simulink model "pack_2s1p_example"  (R2022a)
settings: Solver=VariableStepAuto  StartTime=0.0  StopTime=param.end_time  RelTol=1e-3
values from neighbouring files (symbols this model uses):
  param = table2struct(readtable('settings.csv'))    [run_pybamm_pack.m]
libraries: fl_lib x13, spsParallelRLCBranchLib x8, nesl_utility x5, spsCurrentMeasurementLib x4, spsVoltageMeasurementLib x3, spsControlledVoltageSourceLib x2, spsVariableResistorLib x2, spsControlledCurrentSourceLib x1, spspowerguiLib x1
settings Model: Creator=tom  LastModifiedBy=Vivian
settings SolverCC: AlgebraicLoopSolver=TrustRegion
settings DebuggingCC: UnconnectedInputMsg=warning  UnconnectedOutputMsg=warning  UnconnectedLineMsg=warning  SFMachineParentedDataDiag=warning
settings RTWCC: DLArmComputeVersion=19.05

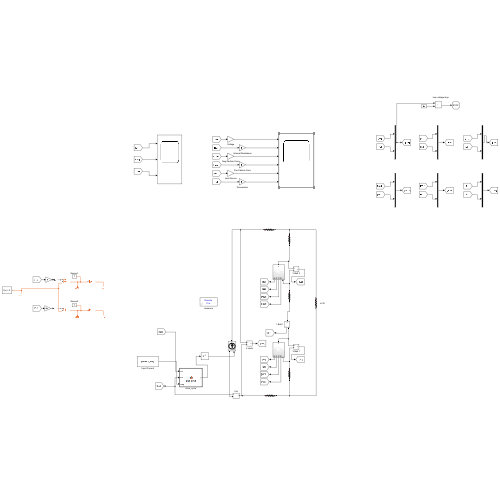
[thumbnail: Simulink's stored preview of the top-level diagram]
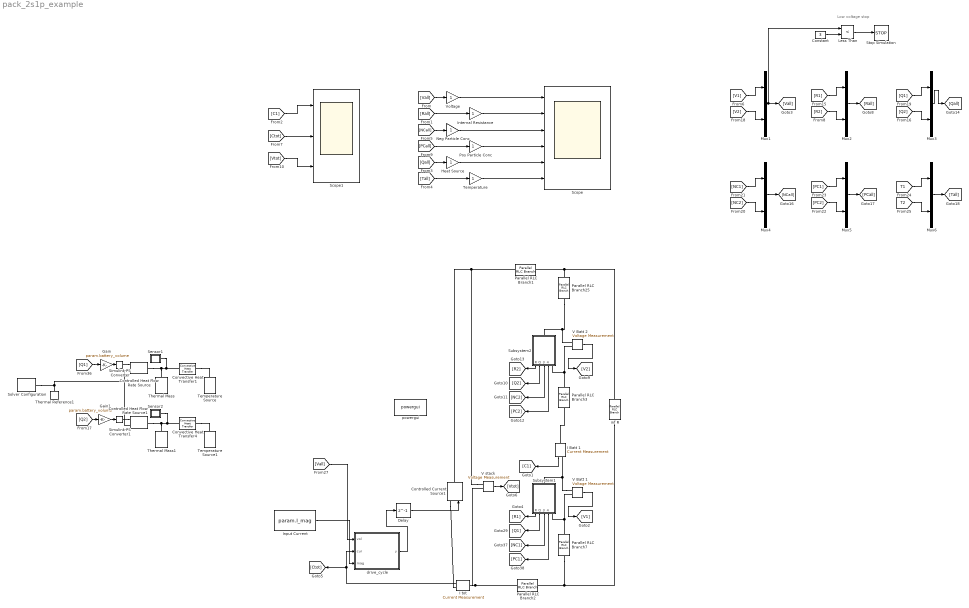
== system pack_2s1p_example ==
  note: Low voltage stop
  Constant : Constant  Value=3
  Controlled Current Source1 : spsControlledCurrentSourceLib/Controlled Current Source  Initialize=on  Source_Type=DC  Amplitude=0  Phase=0  Frequency=0  Measurements=None
  Controlled Heat Flow Rate Source : fl_lib/Thermal/Thermal Sources/Controlled Heat Flow Rate Source
      settings: SourceProductBaseCode=PW,SS,VE
  Controlled Heat Flow Rate Source1 : fl_lib/Thermal/Thermal Sources/Controlled Heat Flow Rate Source
      settings: SourceProductBaseCode=PW,SS,VE
  Convective Heat Transfer1 : fl_lib/Thermal/Thermal Elements/Convective Heat Transfer  area=param.cooled_surface_area m^2  heat_tr_coeff=param.cooling_coefficient W/(m^2 * K)  T_specify=off  T_priority=None  T=0 K  T_nominal_specify=off  T_nominal_unit=K  T_nominal_value=1  Q_specify=off  Q_priority=None  Q=0 W  Q_nominal_specify=off  Q_nominal_unit=W  Q_nominal_value=1
      settings: SourceProductBaseCode=PW,SS,VE
  Convective Heat Transfer4 : fl_lib/Thermal/Thermal Elements/Convective Heat Transfer  area=param.cooled_surface_area m^2  heat_tr_coeff=param.cooling_coefficient W/(m^2 * K)  T_specify=off  T_priority=None  T=0 K  T_nominal_specify=off  T_nominal_unit=K  T_nominal_value=1  Q_specify=off  Q_priority=None  Q=0 W  Q_nominal_specify=off  Q_nominal_unit=W  Q_nominal_value=1
      settings: SourceProductBaseCode=PW,SS,VE
  Delay : Delay  DelayLength=1  InitialCondition=param.I_app
  Gain : Gain  Gain=param.battery_volume
  Gain1 : Gain  Gain=param.battery_volume
  Heat Source : Gain
  I Batt 1 : spsCurrentMeasurementLib/Current Measurement  PhasorSimulation=off  OutputType=Complex  PSBequivalent=0
  I tot : spsCurrentMeasurementLib/Current Measurement  PhasorSimulation=off  OutputType=Complex  PSBequivalent=0
  Input Current : Constant  Value=param.I_mag
  Internal Resistance : Gain
  Less Than : RelationalOperator  Operator=<  OutDataTypeStr=boolean  RndMeth=Simplest  InputSameDT=off
  Mux{1..6} (6 alike) : Mux  Inputs=2
  Neg Particle Conc : Gain
  Parallel RLC Branch1 : spsParallelRLCBranchLib/Parallel RLC Branch  LConnTagsString=a  RConnTagsString=__new0  BranchType=R  Resistance=param.R_connect  Inductance=1e-3  SetiL0=off  InitialCurrent=0  Capacitance=1e-6  Setx0=off  InitialVoltage=0  Measurements=None
  Parallel RLC Branch2 : spsParallelRLCBranchLib/Parallel RLC Branch  LConnTagsString=a  RConnTagsString=__new0  BranchType=R  Resistance=param.R_connect  Inductance=1e-3  SetiL0=off  InitialCurrent=0  Capacitance=1e-6  Setx0=off  InitialVoltage=0  Measurements=None
  Parallel RLC Branch25 : spsParallelRLCBranchLib/Parallel RLC Branch  LConnTagsString=a  RConnTagsString=__new0  BranchType=R  Resistance=param.R_series_top  Inductance=1e-3  SetiL0=off  InitialCurrent=0  Capacitance=1e-6  Setx0=off  InitialVoltage=0  Measurements=None
  Parallel RLC Branch3 : spsParallelRLCBranchLib/Parallel RLC Branch  LConnTagsString=a  RConnTagsString=__new0  BranchType=R  Resistance=param.R_series_mid  Inductance=1e-3  SetiL0=off  InitialCurrent=0  Capacitance=1e-6  Setx0=off  InitialVoltage=0  Measurements=None
  Parallel RLC Branch7 : spsParallelRLCBranchLib/Parallel RLC Branch  LConnTagsString=a  RConnTagsString=__new0  BranchType=R  Resistance=param.R_series_bottom  Inductance=1e-3  SetiL0=off  InitialCurrent=0  Capacitance=1e-6  Setx0=off  InitialVoltage=0  Measurements=None
  Pos Particle Conc : Gain
  Scope : Scope  NumInputPorts=6
  Scope1 : Scope  NumInputPorts=3
  Sensor1 : Subsystem
      mask Display: disp('T')
  Sensor2 : Subsystem
      mask Display: disp('T')
  Simulink-PS Converter : nesl_utility/Simulink-PS Converter  PhysicalDomain=network_engine_domain  SubClassName=ps_input  LeftPortType=input  RightPortType=output  PseudoPeriodic=off  Frequencies=[]  NoiseDistribution=none  NoiseParameters=[]  Unit=1  AffineConversion=off  FilteringAndDerivatives=provide  SimscapeFilterOrder=1  InputFilterTimeConstant=0.001  UdotUserProvided=0
      settings: SourceProductBaseCode=SS,PW,VE
  Simulink-PS Converter1 : nesl_utility/Simulink-PS Converter  PhysicalDomain=network_engine_domain  SubClassName=ps_input  LeftPortType=input  RightPortType=output  PseudoPeriodic=off  Frequencies=[]  NoiseDistribution=none  NoiseParameters=[]  Unit=1  AffineConversion=off  FilteringAndDerivatives=provide  SimscapeFilterOrder=1  InputFilterTimeConstant=0.001  UdotUserProvided=0
      settings: SourceProductBaseCode=SS,PW,VE
  Solver Configuration : nesl_utility/Solver Configuration  PhysicalDomain=network_engine_domain  SubClassName=solver  LeftPortType=input  RightPortType=generic  Tones=[]  Harmonics=[]  SimulateNoise=off  Profile=off  UseLocalSampling=off  EnableSwitchedLinearOptims=on  FrequencyDomain=off  UseCCode=off  RelTol=0.001  AbsTol=1e-06  MinStep=1e-09  ToWorkspace=off  RevertToSquareIcSolve=off  NumHomotopyIterations=100  PhasorMode=off  PhasorModeNumHarmonics=1  IndexReductionMethod=DerivativeReplacement  DoDC=off  ResidualTolerance=1e-09  UseLocalSolver=on  LocalSolverChoice=NE_BACKWARD_EULER_ADVANCER  LocalSolverSampleTime=param.dt  DoFixedCost=on  MaxNonlinIter=3  MaxModeIter=2  ComputeImpulses=off  ImpulseIterations=2  LinearAlgebra=auto  LinearAlgebraNumThread=0  EquationFormulation=NE_TIME_EF  DelaysMemoryBudget=1024  AutomaticFiltering=on  FilteringTimeConstant=0.001  PartitionStorageMethod=AS_NEEDED  PartitionMemoryBudget=1024  PartitionMethod=ROBUST
      settings: SourceProductBaseCode=SS,PW,VE
  Stop Simulation : Stop
  Subsystem1 : Subsystem
  Subsystem2 : Subsystem
  Temperature : Gain
  Temperature Source : fl_lib/Thermal/Thermal Sources/Temperature Source  temperature=param.reference_temperature K
      settings: SourceProductBaseCode=PW,SS,VE
  Temperature Source1 : fl_lib/Thermal/Thermal Sources/Temperature Source  temperature=param.reference_temperature K
      settings: SourceProductBaseCode=PW,SS,VE
  Thermal Mass : fl_lib/Thermal/Thermal Elements/Thermal Mass  mass=param.battery_mass kg  sp_heat=param.Cp J/kg/K  T_specify=on  T_priority=High  T=param.reference_temperature K  T_nominal_specify=off  T_nominal_unit=K  T_nominal_value=1  Q_specify=off  Q_priority=None  Q=0 W  Q_nominal_specify=off  Q_nominal_unit=W  Q_nominal_value=1
      settings: SourceProductBaseCode=PW,SS,VE
  Thermal Mass1 : fl_lib/Thermal/Thermal Elements/Thermal Mass  mass=param.battery_mass kg  sp_heat=param.Cp J/kg/K  T_specify=on  T_priority=High  T=param.reference_temperature K  T_nominal_specify=off  T_nominal_unit=K  T_nominal_value=1  Q_specify=off  Q_priority=None  Q=0 W  Q_nominal_specify=off  Q_nominal_unit=W  Q_nominal_value=1
      settings: SourceProductBaseCode=PW,SS,VE
  Thermal Reference1 : fl_lib/Thermal/Thermal Elements/Thermal Reference
      settings: SourceProductBaseCode=PW,SS,VE
  V Batt 1 : spsVoltageMeasurementLib/Voltage Measurement  PhasorSimulation=off  OutputType=Complex  PSBequivalent=0
  V Batt 2 : spsVoltageMeasurementLib/Voltage Measurement  PhasorSimulation=off  OutputType=Complex  PSBequivalent=0
  V stack : spsVoltageMeasurementLib/Voltage Measurement  PhasorSimulation=off  OutputType=Complex  PSBequivalent=0
  Voltage : Gain
  drive_cycle : MATLAB Function  TreatAsAtomicUnit=on
  inf R : spsParallelRLCBranchLib/Parallel RLC Branch  LConnTagsString=a  RConnTagsString=__new0  BranchType=R  Resistance=100000  Inductance=1e-3  SetiL0=off  InitialCurrent=0  Capacitance=1e-6  Setx0=off  InitialVoltage=0  Measurements=None
  powergui : spspowerguiLib/powergui  Priority=1  SimulationMode=Discrete  SampleTime=param.dt  frequency=60  Iterations=50  frequencyindice=0  Pbase=100e6  ErrMax=1e-4  UnitsV=kV  UnitsW=MW  buscounter=0  FunctionMessages=off  echomessages=off  EnableUseOfTLC=off  CurrentSourceSwitches=off  DisableSnubberDevices=off  DisableRonSwitches=off  DisableVfSwitches=off  DisplayEquations=off  AutomaticDiscreteSolvers=off  SolverType=Tustin/Backward Euler (TBE)  Interpol=off  ExternalGateDelay=off  methode=off  Ts=100  x0status=blocks  SPID=on  SwTol=0  HookPort=off  NonlinearTolerance=1e-4  nMaxIteration=100  ContinueOnMaxIteration=off  RestoreLinks=warning  ResistiveCurrentMeasurement=off  Frange=[0:2:500]  Ylog=off  Xlog=on  ShowGrid=off  save=off  variable=ZData  structure=0  ZoomFFT=off  StartTime=0.0  cycles=1  DisplayStyle=1  fundamental=60  FreqAxis=off  MaxFrequency=1000  frequencyindicesteady=1  RmsSteady=1  display=off
  wires:
  Input Current/1 -> drive_cycle/3(mag)
  [Vall] -> drive_cycle/1(vol)
  drive_cycle/1(y) -> Delay/1
  V stack/1 -> [Vtot]
  V Batt 1/1 -> [V1]
  I Batt 1/1 -> [C1]
  Subsystem1/2(Q) -> [Q1]
  Gain/1 -> Simulink-PS Converter/1
  [Q1] -> Gain/1
  [Vall] -> Voltage/1
  [Rall] -> Internal Resistance/1
  [NCall] -> Neg Particle Conc/1
  [PCall] -> Pos Particle Conc/1
  [Qall] -> Heat Source/1
  [Tall] -> Temperature/1
  [V1] -> Mux1/1
  Mux1/1 -> Less Than/1, [Vall]
  I tot/1 -> [Ctot], drive_cycle/2(cur)
  Subsystem1/1(R) -> [R1]
  Subsystem2/1(R) -> [R2]
  Subsystem2/2(Q) -> [Q2]
  V Batt 2/1 -> [V2]
  [Q2] -> Gain1/1
  Gain1/1 -> Simulink-PS Converter1/1
  [V2] -> Mux1/2
  Delay/1 -> Controlled Current Source1/1
  [R2] -> Mux2/2
  Mux2/1 -> [Rall]
  [R1] -> Mux2/1
  [Q2] -> Mux3/2
  Mux3/1 -> [Qall]
  [Q1] -> Mux3/1
  [NC2] -> Mux4/2
  Mux4/1 -> [NCall]
  [NC1] -> Mux4/1
  Mux5/1 -> [PCall]
  [PC2] -> Mux5/2
  [PC1] -> Mux5/1
  [T1] -> Mux6/1
  Mux6/1 -> [Tall]
  [T2] -> Mux6/2
  Voltage/1 -> Scope/1
  Internal Resistance/1 -> Scope/2
  Neg Particle Conc/1 -> Scope/3
  Pos Particle Conc/1 -> Scope/4
  Heat Source/1 -> Scope/5
  Temperature/1 -> Scope/6
  Subsystem2/3(nc) -> [NC2]
  Subsystem2/4(pc) -> [PC2]
  Subsystem1/3(nc) -> [NC1]
  Subsystem1/4(pc) -> [PC1]
  [C1] -> Scope1/1
  [Ctot] -> Scope1/2
  [Vtot] -> Scope1/3
  Less Than/1 -> Stop Simulation/1
  Constant/1 -> Less Than/2
  connections:
  Parallel RLC Branch25/LConn1 -- inf R/LConn1 -- Parallel RLC Branch1/RConn1
  V stack/LConn1 -- Controlled Current Source1/RConn1 -- Parallel RLC Branch1/LConn1
  Subsystem1/RConn1 -- V Batt 1/LConn2 -- Parallel RLC Branch7/LConn1
  V Batt 1/LConn1 -- I Batt 1/RConn1 -- Subsystem1/LConn1
  V stack/LConn2 -- Parallel RLC Branch2/LConn1 -- I tot/LConn1
  Parallel RLC Branch7/RConn1 -- Parallel RLC Branch2/RConn1 -- inf R/RConn1
  Thermal Mass/LConn1 -- Sensor1/LConn1 -- Convective Heat Transfer1/LConn1 -- Controlled Heat Flow Rate Source/LConn1
  Simulink-PS Converter/RConn1 -- Controlled Heat Flow Rate Source/RConn1
  Thermal Reference1/LConn1 -- Solver Configuration/RConn1 -- Controlled Heat Flow Rate Source1/RConn2 -- Controlled Heat Flow Rate Source/RConn2
  Controlled Current Source1/LConn1 -- I tot/RConn1
  Subsystem2/RConn1 -- Parallel RLC Branch3/LConn1 -- V Batt 2/LConn2
  Subsystem2/LConn1 -- Parallel RLC Branch25/RConn1 -- V Batt 2/LConn1
  I Batt 1/LConn1 -- Parallel RLC Branch3/RConn1
  Thermal Mass1/LConn1 -- Sensor2/LConn1 -- Convective Heat Transfer4/LConn1 -- Controlled Heat Flow Rate Source1/LConn1
  Simulink-PS Converter1/RConn1 -- Controlled Heat Flow Rate Source1/RConn1
  Convective Heat Transfer4/RConn1 -- Temperature Source1/LConn1
  Convective Heat Transfer1/RConn1 -- Temperature Source/LConn1

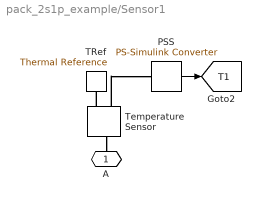
== system pack_2s1p_example/Sensor1 ==
  PSS : nesl_utility/PS-Simulink Converter  PhysicalDomain=network_engine_domain  SubClassName=ps_output  LeftPortType=input  RightPortType=output  PseudoPeriodic=off  Frequencies=[]  VectorFormat=1-D array  Unit=1  AffineConversion=off
      settings: SourceProductBaseCode=SS,PW,VE
  TRef : fl_lib/Thermal/Thermal Elements/Thermal Reference
      settings: SourceProductBaseCode=PW,SS,VE
  Temperature Sensor : fl_lib/Thermal/Thermal Sensors/Temperature Sensor
      settings: SourceProductBaseCode=PW,SS,VE
  A : PMIOPort  Side=Left
  tag scope: T1=global
  wires:
  PSS/1 -> [T1]
  connections:
  Temperature Sensor/RConn2 -- PSS/LConn1
  Temperature Sensor/RConn1 -- TRef/LConn1
  Temperature Sensor/LConn1 -- A/RConn1

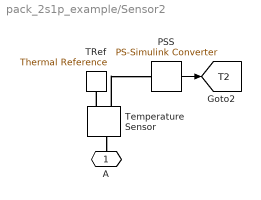
== system pack_2s1p_example/Sensor2 ==
  PSS : nesl_utility/PS-Simulink Converter  PhysicalDomain=network_engine_domain  SubClassName=ps_output  LeftPortType=input  RightPortType=output  PseudoPeriodic=off  Frequencies=[]  VectorFormat=1-D array  Unit=1  AffineConversion=off
      settings: SourceProductBaseCode=SS,PW,VE
  TRef : fl_lib/Thermal/Thermal Elements/Thermal Reference
      settings: SourceProductBaseCode=PW,SS,VE
  Temperature Sensor : fl_lib/Thermal/Thermal Sensors/Temperature Sensor
      settings: SourceProductBaseCode=PW,SS,VE
  A : PMIOPort  Side=Left
  tag scope: T2=global
  wires:
  PSS/1 -> [T2]
  connections:
  Temperature Sensor/LConn1 -- A/RConn1
  Temperature Sensor/RConn1 -- TRef/LConn1
  Temperature Sensor/RConn2 -- PSS/LConn1

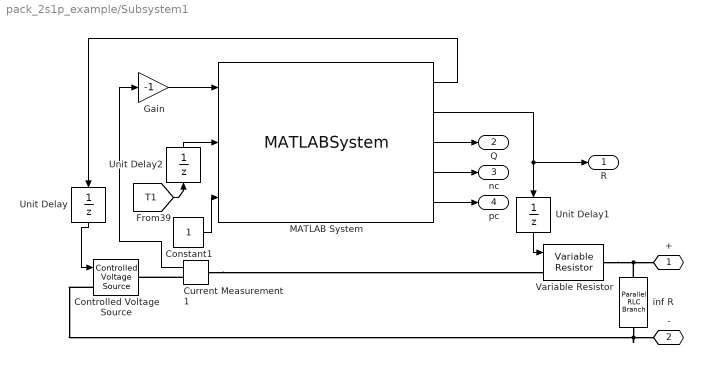
== system pack_2s1p_example/Subsystem1 ==
  Constant1 : Constant
  Controlled Voltage Source : spsControlledVoltageSourceLib/Controlled Voltage Source  Initialize=on  Source_Type=AC  Amplitude=0  Phase=0  Frequency=0  Measurements=None
  Current Measurement1 : spsCurrentMeasurementLib/Current Measurement  PhasorSimulation=off  OutputType=Complex  PSBequivalent=0
  Gain : Gain  Gain=-1
  MATLAB System : MATLABSystem  System=casadi_bat  SimulateUsing=Interpreted execution
      mask Type: casadi_bat
      mask Display:
      | disp('casadi_bat');
      | port_label('input',1,'current');
      | port_label('input',2,'temperature');
      | port_label('input',3,'soc_init');
      | port_label('output',1,'ocp');
      | port_label('output',2,'internal_resistance');
      | port_label('output',3,'heating');
      | port_label('output',4,'neg_conc');
      | port_label('output',5,'pos_conc');
  Unit Delay : UnitDelay  InitialCondition=param.ocv_init  SampleTime=-1  HasFrameUpgradeWarning=on
  Unit Delay1 : UnitDelay  InitialCondition=param.r_int_init  SampleTime=-1  HasFrameUpgradeWarning=on
  Unit Delay2 : UnitDelay  InitialCondition=param.t_init  SampleTime=-1  HasFrameUpgradeWarning=on
  Variable Resistor : spsVariableResistorLib/Variable Resistor  Rabsmin=1e-3
      settings: SourceProductBaseCode=PS
  inf R : spsParallelRLCBranchLib/Parallel RLC Branch  LConnTagsString=a  RConnTagsString=__new0  BranchType=R  Resistance=100000  Inductance=1e-3  SetiL0=off  InitialCurrent=0  Capacitance=1e-6  Setx0=off  InitialVoltage=0  Measurements=None
  + : PMIOPort  Tag=PMCPort  Side=Left
  - : PMIOPort  Tag=PMCPort  Port=2  Side=Right
  R : Outport  VectorParamsAs1DForOutWhenUnconnected=off
  Q : Outport  Port=2  VectorParamsAs1DForOutWhenUnconnected=off
  nc : Outport  Port=3  VectorParamsAs1DForOutWhenUnconnected=off
  pc : Outport  Port=4  VectorParamsAs1DForOutWhenUnconnected=off
  wires:
  Gain/1 -> MATLAB System/1
  MATLAB System/1 -> Unit Delay/1
  Current Measurement1/1 -> Gain/1
  Unit Delay/1 -> Controlled Voltage Source/1
  MATLAB System/2 -> R/1, Unit Delay1/1
  Unit Delay1/1 -> Variable Resistor/1
  MATLAB System/3 -> Q/1
  Unit Delay2/1 -> MATLAB System/2
  [T1] -> Unit Delay2/1
  MATLAB System/5 -> pc/1
  MATLAB System/4 -> nc/1
  Constant1/1 -> MATLAB System/3
  connections:
  Current Measurement1/RConn1 -- Controlled Voltage Source/RConn1
  Controlled Voltage Source/LConn1 -- inf R/RConn1 -- -/RConn1
  Current Measurement1/LConn1 -- Variable Resistor/LConn1
  Variable Resistor/RConn1 -- inf R/LConn1 -- +/RConn1

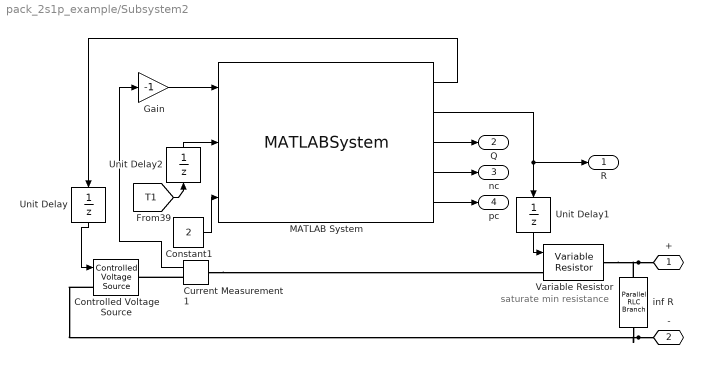
== system pack_2s1p_example/Subsystem2 ==
  note: saturate min resistance
  Constant1 : Constant  Value=2
  Controlled Voltage Source : spsControlledVoltageSourceLib/Controlled Voltage Source  Initialize=on  Source_Type=AC  Amplitude=0  Phase=0  Frequency=0  Measurements=None
  Current Measurement1 : spsCurrentMeasurementLib/Current Measurement  PhasorSimulation=off  OutputType=Complex  PSBequivalent=0
  Gain : Gain  Gain=-1
  MATLAB System : MATLABSystem  System=casadi_bat  SimulateUsing=Interpreted execution
      mask Type: casadi_bat
      mask Display:
      | disp('casadi_bat');
      | port_label('input',1,'current');
      | port_label('input',2,'temperature');
      | port_label('input',3,'soc_init');
      | port_label('output',1,'ocp');
      | port_label('output',2,'internal_resistance');
      | port_label('output',3,'heating');
      | port_label('output',4,'neg_conc');
      | port_label('output',5,'pos_conc');
  Unit Delay : UnitDelay  InitialCondition=param.ocv_init  SampleTime=-1  HasFrameUpgradeWarning=on
  Unit Delay1 : UnitDelay  InitialCondition=param.r_int_init  SampleTime=-1  HasFrameUpgradeWarning=on
  Unit Delay2 : UnitDelay  InitialCondition=param.t_init  SampleTime=-1  HasFrameUpgradeWarning=on
  Variable Resistor : spsVariableResistorLib/Variable Resistor  Rabsmin=1e-3
      settings: SourceProductBaseCode=PS
  inf R : spsParallelRLCBranchLib/Parallel RLC Branch  LConnTagsString=a  RConnTagsString=__new0  BranchType=R  Resistance=100000  Inductance=1e-3  SetiL0=off  InitialCurrent=0  Capacitance=1e-6  Setx0=off  InitialVoltage=0  Measurements=None
  + : PMIOPort  Tag=PMCPort  Side=Left
  - : PMIOPort  Tag=PMCPort  Port=2  Side=Right
  R : Outport  VectorParamsAs1DForOutWhenUnconnected=off
  Q : Outport  Port=2  VectorParamsAs1DForOutWhenUnconnected=off
  nc : Outport  Port=3  VectorParamsAs1DForOutWhenUnconnected=off
  pc : Outport  Port=4  VectorParamsAs1DForOutWhenUnconnected=off
  wires:
  MATLAB System/4 -> nc/1
  MATLAB System/5 -> pc/1
  [T1] -> Unit Delay2/1
  Unit Delay2/1 -> MATLAB System/2
  MATLAB System/3 -> Q/1
  Unit Delay1/1 -> Variable Resistor/1
  MATLAB System/2 -> Unit Delay1/1, R/1
  Unit Delay/1 -> Controlled Voltage Source/1
  Current Measurement1/1 -> Gain/1
  MATLAB System/1 -> Unit Delay/1
  Gain/1 -> MATLAB System/1
  Constant1/1 -> MATLAB System/3
  connections:
  +/RConn1 -- inf R/LConn1 -- Variable Resistor/RConn1
  Current Measurement1/LConn1 -- Variable Resistor/LConn1
  -/RConn1 -- inf R/RConn1 -- Controlled Voltage Source/LConn1
  Current Measurement1/RConn1 -- Controlled Voltage Source/RConn1

== matlab function pack_2s1p_example/drive_cycle ==
  data: y output; vol input; cur input; mag input
function y  = drive_cycle(vol, cur, mag)

y = 0;

status=sign(cur);
if min(vol)<=2.5
    if status==-1
        status=1; % charge
    end
elseif max(vol)>=4.2
    if status==1
        status=-1;% discharge
    end
end

if status==-1
    y=-mag;
else
    y=mag;
end
